simulink model "Battery_Soc"  (R2021b)
settings: Solver=VariableStepAuto  StartTime=0.0  StopTime=sim_time  RelTol=1e-3
values from neighbouring files (symbols this model uses):
  cn = (2.3*3600)    (= 8280)    [EV_Battery_Mod_MATSCRIPT.m]
  i = 2.3    [EV_Battery_Mod_MATSCRIPT.m]
  ocv = data(:,2)    [EV_Battery_Mod_MATSCRIPT.m]
  r_discharge = data(:,4)    [EV_Battery_Mod_MATSCRIPT.m]
  soc = data(:,1)    [EV_Battery_Mod_MATSCRIPT.m]
settings Model: Creator=Vansh  LastModifiedBy=Vansh

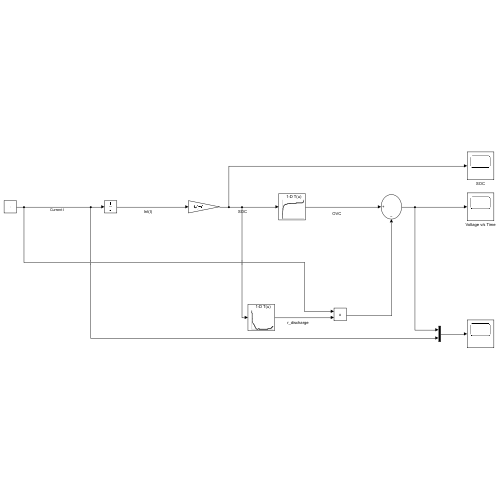
[thumbnail: Simulink's stored preview of the top-level diagram]
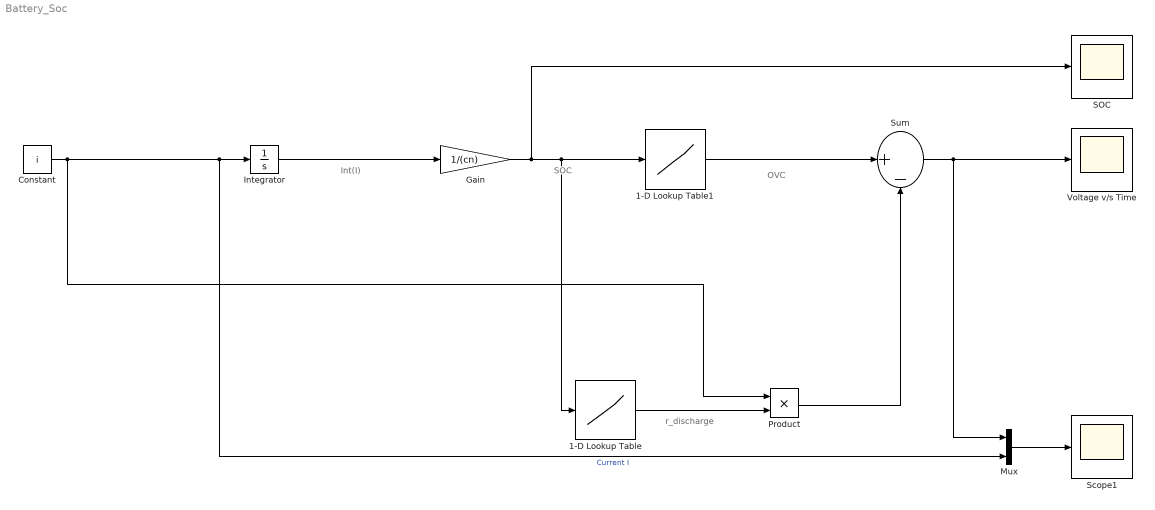
== system Battery_Soc ==
  note: Int(I)
  note: SOC
  note: OVC
  note: r_discharge
  1-D Lookup Table : Lookup_n-D  NumberOfTableDimensions=1  BreakpointsForDimension1=soc  Table=r_discharge  InternalRulePriority=Speed  RndMeth=Simplest  InputSameDT=on
  1-D Lookup Table1 : Lookup_n-D  NumberOfTableDimensions=1  BreakpointsForDimension1=soc  Table=ocv  InternalRulePriority=Speed  RndMeth=Simplest  InputSameDT=on
  Constant : Constant  Value=i
  Gain : Gain  Gain=1/(cn)
  Integrator : Integrator
  Mux : Mux  Inputs=2
  Product : Product
  SOC : Scope
  Scope1 : Scope
  Sum : Sum  Inputs=|+-
  Voltage v/s Time : Scope
  wires:
  Constant/1 -> Product/1, Mux/2, Integrator/1  "Current I"
  Integrator/1 -> Gain/1
  Gain/1 -> SOC/1, 1-D Lookup Table/1, 1-D Lookup Table1/1
  1-D Lookup Table1/1 -> Sum/1
  1-D Lookup Table/1 -> Product/2
  Product/1 -> Sum/2
  Sum/1 -> Mux/1, Voltage v/s Time/1
  Mux/1 -> Scope1/1
